simulink model "ADMIRE"  (R2021b)
settings: Solver=ode4  StartTime=0.0  StopTime=100  FixedStep=1e-2  RelTol=1e-3
undefined symbols (not defined in the file or in its folder): admireDB, Earth, WGS84
libraries: simulink_extras x112, simulink x27, aerolibutil x4, dspsigops x4, aerolibfltsims x3, sharedtransform x2, aerolibtransform2 x2, aerolibatmos2 x1, matrix_library x1, sharedutil x1, aerolibanimutils x1, vrlib x1
(part 9 of 15)

== system ADMIRE/Aircraft/Aerodynamics/CentripetalForceCoefficient/MachRegion1/Ccbde/Ccbde_ ==
  angleOfSideslip_deg : Inport
  dEI : Inport  Port=2
  angleOfAttack_deg : Inport  Port=3
  eieff : Inport  Port=4
  dEY : Inport  Port=5
  eoeff : Inport  Port=6
  Abs : Abs
  CCDEB_ALFA_DE_BETA : Lookup_n-D  NumberOfTableDimensions=3  BreakpointsForDimension1=admireDB.aerodata_asym_ext.CCDEB.breakpoints.ALFA  BreakpointsForDimension2=admireDB.aerodata_asym_ext.CCDEB.breakpoints.DE  BreakpointsForDimension3=admireDB.aerodata_asym_ext.CCDEB.breakpoints.BETA  Table=admireDB.aerodata_asym_ext.CCDEB.newTable  ExtrapMethod=Clip  InternalRulePriority=Speed  RndMeth=Simplest  InputSameDT=on
      settings: InputPortMap=u0,u1,u2
  CCDEB_ALFA_DE_BETA1 : Lookup_n-D  NumberOfTableDimensions=3  BreakpointsForDimension1=admireDB.aerodata_asym_ext.CCDEB.breakpoints.ALFA  BreakpointsForDimension2=admireDB.aerodata_asym_ext.CCDEB.breakpoints.DE  BreakpointsForDimension3=admireDB.aerodata_asym_ext.CCDEB.breakpoints.BETA  Table=admireDB.aerodata_asym_ext.CCDEB.newTable  ExtrapMethod=Clip  InternalRulePriority=Speed  RndMeth=Simplest  InputSameDT=on
      settings: InputPortMap=u0,u1,u2
  Product : Product  Inputs=**
  Product1 : Product  Inputs=**
  Product2 : Product  Inputs=**
  Sign : Signum
  Sum : Sum  Inputs=|++
  Ccbde : Outport
  wires:
  Abs/1 -> CCDEB_ALFA_DE_BETA1/3, CCDEB_ALFA_DE_BETA/3
  angleOfSideslip_deg/1 -> Sign/1, Abs/1
  Product2/1 -> Ccbde/1
  Sign/1 -> Product2/1
  Sum/1 -> Product2/2
  Product1/1 -> Sum/2
  Product/1 -> Sum/1
  CCDEB_ALFA_DE_BETA1/1 -> Product1/1
  eoeff/1 -> Product1/2
  dEY/1 -> CCDEB_ALFA_DE_BETA1/2
  CCDEB_ALFA_DE_BETA/1 -> Product/1
  eieff/1 -> Product/2
  dEI/1 -> CCDEB_ALFA_DE_BETA/2
  angleOfAttack_deg/1 -> CCDEB_ALFA_DE_BETA1/1, CCDEB_ALFA_DE_BETA/1

== system ADMIRE/Aircraft/Aerodynamics/CentripetalForceCoefficient/MachRegion1/Ccbdle/Ccbdle_ ==
  dLE : Inport
  angleOfSideslip_deg : Inport  Port=2
  angleOfAttack_deg : Inport  Port=3
  Abs : Abs
  CCDLEB_ALFA_BETA_DLE : Lookup_n-D  NumberOfTableDimensions=3  BreakpointsForDimension1=admireDB.aerodata_asym_ext.CCDLEB.breakpoints.ALFA  BreakpointsForDimension2=admireDB.aerodata_asym_ext.CCDLEB.breakpoints.BETA  BreakpointsForDimension3=admireDB.aerodata_asym_ext.CCDLEB.breakpoints.DLE  Table=admireDB.aerodata_asym_ext.CCDLEB.newTable  ExtrapMethod=Clip  InternalRulePriority=Speed  RndMeth=Simplest  InputSameDT=on
      settings: InputPortMap=u0,u1,u2
  Product : Product  Inputs=**
  Sign : Signum
  Ccbdle : Outport
  wires:
  Product/1 -> Ccbdle/1
  Sign/1 -> Product/2
  CCDLEB_ALFA_BETA_DLE/1 -> Product/1
  Abs/1 -> CCDLEB_ALFA_BETA_DLE/2
  angleOfAttack_deg/1 -> CCDLEB_ALFA_BETA_DLE/1
  angleOfSideslip_deg/1 -> Sign/1, Abs/1
  dLE/1 -> CCDLEB_ALFA_BETA_DLE/3

== system ADMIRE/Aircraft/Aerodynamics/CentripetalForceCoefficient/MachRegion1/Ccbdn/Ccbdn_ ==
  angleOfSideslip_deg : Inport
  dN : Inport  Port=2
  angleOfAttack_deg : Inport  Port=3
  Abs : Abs
  CCDNB_ALFA_DN_BETA : Lookup_n-D  NumberOfTableDimensions=3  BreakpointsForDimension1=admireDB.aerodata_asym_ext.CCDNB.breakpoints.ALFA  BreakpointsForDimension2=admireDB.aerodata_asym_ext.CCDNB.breakpoints.DN  BreakpointsForDimension3=admireDB.aerodata_asym_ext.CCDNB.breakpoints.BETA  Table=admireDB.aerodata_asym_ext.CCDNB.newTable  ExtrapMethod=Clip  InternalRulePriority=Speed  RndMeth=Simplest  InputSameDT=on
      settings: InputPortMap=u0,u1,u2
  Product : Product  Inputs=**
  Sign : Signum
  Ccbdn : Outport
  wires:
  Abs/1 -> CCDNB_ALFA_DN_BETA/3
  angleOfAttack_deg/1 -> CCDNB_ALFA_DN_BETA/1
  Product/1 -> Ccbdn/1
  Sign/1 -> Product/2
  CCDNB_ALFA_DN_BETA/1 -> Product/1
  dN/1 -> CCDNB_ALFA_DN_BETA/2
  angleOfSideslip_deg/1 -> Abs/1, Sign/1

== system ADMIRE/Aircraft/Aerodynamics/CentripetalForceCoefficient/MachRegion1/Ccbeta/Ccbeta_ ==
  angleOfSideslip_deg : Inport
  angleOfAttack_deg : Inport  Port=2
  qacorr : Inport  Port=3
  mach_nd : Inport  Port=4
  Abs : Abs
  CCBAL_BETA_ALFA : Lookup_n-D  BreakpointsForDimension1=admireDB.aerodata_asym_ext.CCBAL.breakpoints.ALFA  BreakpointsForDimension2=admireDB.aerodata_asym_ext.CCBAL.breakpoints.BETA  BreakpointsForDimension3=[5, 7]  Table=admireDB.aerodata_asym_ext.CCBAL.newTable  ExtrapMethod=Clip  InternalRulePriority=Speed  RndMeth=Simplest  InputSameDT=on
      settings: InputPortMap=u0,u1
  CCEB_QA_M : Lookup_n-D  BreakpointsForDimension1=admireDB.aerodata_asym_ext.CCEB.breakpoints.M  BreakpointsForDimension2=admireDB.aerodata_asym_ext.CCEB.breakpoints.QA  BreakpointsForDimension3=[5, 7]  Table=admireDB.aerodata_asym_ext.CCEB.newTable  ExtrapMethod=Clip  InternalRulePriority=Speed  RndMeth=Simplest  InputSameDT=on
      settings: InputPortMap=u0,u1
  Product : Product  Inputs=***
  Sign : Signum
  Ccbeta : Outport
  wires:
  Product/1 -> Ccbeta/1
  Sign/1 -> Product/1
  CCBAL_BETA_ALFA/1 -> Product/2
  CCEB_QA_M/1 -> Product/3
  Abs/1 -> CCBAL_BETA_ALFA/2
  angleOfSideslip_deg/1 -> Abs/1, Sign/1
  angleOfAttack_deg/1 -> CCBAL_BETA_ALFA/1
  qacorr/1 -> CCEB_QA_M/2
  mach_nd/1 -> CCEB_QA_M/1

== system ADMIRE/Aircraft/Aerodynamics/CentripetalForceCoefficient/MachRegion1/Ccbetad/Ccbetad_ ==
  angleOfAttack_deg : Inport
  betad : Inport  Port=2
  CCBDL_ALFA : Lookup_n-D  NumberOfTableDimensions=1  BreakpointsForDimension1=admireDB.aerodata_asym_ext.CCBDL.breakpoints.ALFA  BreakpointsForDimension3=[5, 7]  Table=admireDB.aerodata_asym_ext.CCBDL.newTable  ExtrapMethod=Clip  InternalRulePriority=Speed  RndMeth=Simplest  InputSameDT=on
  Product : Product
  Ccbetad : Outport
  wires:
  Product/1 -> Ccbetad/1
  betad/1 -> Product/2
  CCBDL_ALFA/1 -> Product/1
  angleOfAttack_deg/1 -> CCBDL_ALFA/1

== system ADMIRE/Aircraft/Aerodynamics/CentripetalForceCoefficient/MachRegion1/Ccblg/Ccblg_ ==
  dLG : Inport
  angleOfAttack_deg : Inport  Port=2
  angleOfSideslip_deg : Inport  Port=3
  CCBLST_NG_DOOR_ALFA : Lookup_n-D  BreakpointsForDimension1=admireDB.aerodata_asym_ext.CCBLST.breakpoints.ALFA  BreakpointsForDimension2=admireDB.aerodata_asym_ext.CCBLST.breakpoints.NG_DOOR  BreakpointsForDimension3=[5, 7]  Table=admireDB.aerodata_asym_ext.CCBLST.newTable  ExtrapMethod=Clip  InternalRulePriority=Speed  RndMeth=Simplest  InputSameDT=on
      settings: InputPortMap=u0,u1
  Degrees to Radians : simulink_extras/Transformations/Degrees to Radians
  Product : Product  Inputs=***
  Ccblg : Outport
  wires:
  Product/1 -> Ccblg/1
  Degrees to Radians/1 -> Product/2
  angleOfSideslip_deg/1 -> Degrees to Radians/1
  CCBLST_NG_DOOR_ALFA/1 -> Product/1
  dLG/1 -> Product/3, CCBLST_NG_DOOR_ALFA/2
  angleOfAttack_deg/1 -> CCBLST_NG_DOOR_ALFA/1

== system ADMIRE/Aircraft/Aerodynamics/CentripetalForceCoefficient/MachRegion1/Ccdai/Ccdai_ ==
  dAI : Inport
  angleOfAttack_deg : Inport  Port=2
  dEI : Inport  Port=3
  eieff : Inport  Port=4
  qacorr : Inport  Port=5
  mach_nd : Inport  Port=6
  Abs : Abs
  CCDAAL_DA_ALFA : Lookup_n-D  BreakpointsForDimension1=admireDB.aerodata_asym_ext.CCDAAL.breakpoints.ALFA  BreakpointsForDimension2=admireDB.aerodata_asym_ext.CCDAAL.breakpoints.DA  BreakpointsForDimension3=[5, 7]  Table=admireDB.aerodata_asym_ext.CCDAAL.newTable  ExtrapMethod=Clip  InternalRulePriority=Speed  RndMeth=Simplest  InputSameDT=on
      settings: InputPortMap=u0,u1
  CCDAL_DE_ALFA : Lookup_n-D  BreakpointsForDimension1=admireDB.aerodata_asym_ext.CCDAL.breakpoints.ALFA  BreakpointsForDimension2=admireDB.aerodata_asym_ext.CCDAL.breakpoints.DE  BreakpointsForDimension3=[5, 7]  Table=admireDB.aerodata_asym_ext.CCDAL.newTable  ExtrapMethod=Clip  InternalRulePriority=Speed  RndMeth=Simplest  InputSameDT=on
      settings: InputPortMap=u0,u1
  CCDAL_DE_ALFA_1 : Lookup_n-D  BreakpointsForDimension1=admireDB.aerodata_asym_ext.CCDAL.breakpoints.ALFA  BreakpointsForDimension2=admireDB.aerodata_asym_ext.CCDAL.breakpoints.DE  BreakpointsForDimension3=[5, 7]  Table=admireDB.aerodata_asym_ext.CCDAL.newTable  ExtrapMethod=Clip  InternalRulePriority=Speed  RndMeth=Simplest  InputSameDT=on
      settings: InputPortMap=u0,u1
  CCEDAI_QA_M : Lookup_n-D  BreakpointsForDimension1=admireDB.aerodata_asym_ext.CCEDAI.breakpoints.M  BreakpointsForDimension2=admireDB.aerodata_asym_ext.CCEDAI.breakpoints.QA  BreakpointsForDimension3=[5, 7]  Table=admireDB.aerodata_asym_ext.CCEDAI.newTable  ExtrapMethod=Clip  InternalRulePriority=Speed  RndMeth=Simplest  InputSameDT=on
      settings: InputPortMap=u0,u1
  Degrees to Radians : simulink_extras/Transformations/Degrees to Radians
  Product : Product  Inputs=**
  Product1 : Product  Inputs=**
  Product2 : Product  Inputs=3
  Sign : Signum
  Sum : Sum  Inputs=|++
  Sum1 : Sum  Inputs=|+-
  dE_cnst : Constant  Value=0.0
  Ccdai : Outport
  wires:
  Sum1/1 -> Product1/2
  Product2/1 -> Ccdai/1
  CCEDAI_QA_M/1 -> Product2/3
  qacorr/1 -> CCEDAI_QA_M/2
  mach_nd/1 -> CCEDAI_QA_M/1
  Sum/1 -> Product2/1
  eieff/1 -> Product2/2
  Product1/1 -> Sum/2
  Degrees to Radians/1 -> Product1/1
  CCDAL_DE_ALFA_1/1 -> Sum1/2
  CCDAL_DE_ALFA/1 -> Sum1/1
  angleOfAttack_deg/1 -> CCDAL_DE_ALFA/1, CCDAL_DE_ALFA_1/1, CCDAAL_DA_ALFA/1
  dEI/1 -> CCDAL_DE_ALFA/2
  dE_cnst/1 -> CCDAL_DE_ALFA_1/2
  Product/1 -> Sum/1
  Abs/1 -> CCDAAL_DA_ALFA/2
  Sign/1 -> Product/1
  CCDAAL_DA_ALFA/1 -> Product/2
  dAI/1 -> Sign/1, Abs/1, Degrees to Radians/1

== system ADMIRE/Aircraft/Aerodynamics/CentripetalForceCoefficient/MachRegion1/Ccdaib/Ccdaib_ ==
  angleOfAttack_deg : Inport
  dAI : Inport  Port=2
  angleOfSideslip_deg : Inport  Port=3
  eieff : Inport  Port=4
  Abs : Abs
  Abs1 : Abs
  Abs2 : Abs
  CCDABAL_ALFA : Lookup_n-D  NumberOfTableDimensions=1  BreakpointsForDimension1=admireDB.aerodata_asym_ext.CCDABAL.breakpoints.ALFA  BreakpointsForDimension3=[5, 7]  Table=admireDB.aerodata_asym_ext.CCDABAL.newTable  ExtrapMethod=Clip  InternalRulePriority=Speed  RndMeth=Simplest  InputSameDT=on
  Constant : Constant  Value=30
  Constant1 : Constant  Value=20
  Product : Product  Inputs=**/*/*
  Ccdaib : Outport
  wires:
  Abs2/1 -> CCDABAL_ALFA/1
  Constant1/1 -> Product/5
  Abs1/1 -> Product/4
  angleOfSideslip_deg/1 -> Abs1/1
  Constant/1 -> Product/3
  Abs/1 -> Product/2
  CCDABAL_ALFA/1 -> Product/1
  Product/1 -> Ccdaib/1
  angleOfAttack_deg/1 -> Abs2/1
  dAI/1 -> Abs/1
  eieff/1 -> Product/6

== system ADMIRE/Aircraft/Aerodynamics/CentripetalForceCoefficient/MachRegion1/Ccday/Ccday_ ==
  dAY : Inport
  angleOfAttack_deg : Inport  Port=2
  dEY : Inport  Port=3
  eoeff : Inport  Port=4
  qacorr : Inport  Port=5
  mach_nd : Inport  Port=6
  Abs : Abs
  CCDAAL_DA_ALFA : Lookup_n-D  BreakpointsForDimension1=admireDB.aerodata_asym_ext.CCDAAL.breakpoints.ALFA  BreakpointsForDimension2=admireDB.aerodata_asym_ext.CCDAAL.breakpoints.DA  BreakpointsForDimension3=[5, 7]  Table=admireDB.aerodata_asym_ext.CCDAAL.newTable  ExtrapMethod=Clip  InternalRulePriority=Speed  RndMeth=Simplest  InputSameDT=on
      settings: InputPortMap=u0,u1
  CCDAL_DE_ALFA : Lookup_n-D  BreakpointsForDimension1=admireDB.aerodata_asym_ext.CCDAL.breakpoints.ALFA  BreakpointsForDimension2=admireDB.aerodata_asym_ext.CCDAL.breakpoints.DE  BreakpointsForDimension3=[5, 7]  Table=admireDB.aerodata_asym_ext.CCDAL.newTable  ExtrapMethod=Clip  InternalRulePriority=Speed  RndMeth=Simplest  InputSameDT=on
      settings: InputPortMap=u0,u1
  CCDAL_DE_ALFA_1 : Lookup_n-D  BreakpointsForDimension1=admireDB.aerodata_asym_ext.CCDAL.breakpoints.ALFA  BreakpointsForDimension2=admireDB.aerodata_asym_ext.CCDAL.breakpoints.DE  BreakpointsForDimension3=[5, 7]  Table=admireDB.aerodata_asym_ext.CCDAL.newTable  ExtrapMethod=Clip  InternalRulePriority=Speed  RndMeth=Simplest  InputSameDT=on
      settings: InputPortMap=u0,u1
  CCEDAY_QA_M : Lookup_n-D  BreakpointsForDimension1=admireDB.aerodata_asym_ext.CCEDAY.breakpoints.M  BreakpointsForDimension2=admireDB.aerodata_asym_ext.CCEDAY.breakpoints.QA  BreakpointsForDimension3=[5, 7]  Table=admireDB.aerodata_asym_ext.CCEDAY.newTable  ExtrapMethod=Clip  InternalRulePriority=Speed  RndMeth=Simplest  InputSameDT=on
      settings: InputPortMap=u0,u1
  Degrees to Radians : simulink_extras/Transformations/Degrees to Radians
  Product : Product  Inputs=**
  Product1 : Product  Inputs=**
  Product2 : Product
  Product3 : Product
  Sign : Signum
  Sum : Sum  Inputs=|++
  Sum1 : Sum  Inputs=|++
  Sum2 : Sum  Inputs=|+-
  dE_cnst : Constant  Value=0.0
  Ccday : Outport
  wires:
  Sum2/1 -> Product1/2
  CCDAL_DE_ALFA_1/1 -> Sum2/2
  CCDAL_DE_ALFA/1 -> Sum2/1
  CCEDAY_QA_M/1 -> Product3/2
  Product2/1 -> Sum1/1
  Sum1/1 -> Ccday/1
  dAY/1 -> Abs/1, Degrees to Radians/1, Sign/1
  CCDAAL_DA_ALFA/1 -> Product/2
  Sign/1 -> Product/1
  Abs/1 -> CCDAAL_DA_ALFA/2
  Product/1 -> Sum/1
  dE_cnst/1 -> CCDAL_DE_ALFA_1/2
  dEY/1 -> CCDAL_DE_ALFA/2
  angleOfAttack_deg/1 -> CCDAL_DE_ALFA/1, CCDAL_DE_ALFA_1/1, CCDAAL_DA_ALFA/1
  Degrees to Radians/1 -> Product1/1, Product3/1
  Product1/1 -> Sum/2
  eoeff/1 -> Product2/2
  Sum/1 -> Product2/1
  mach_nd/1 -> CCEDAY_QA_M/1
  qacorr/1 -> CCEDAY_QA_M/2
  Product3/1 -> Sum1/2

== system ADMIRE/Aircraft/Aerodynamics/CentripetalForceCoefficient/MachRegion1/Ccdayb/Ccdayb_ ==
  angleOfAttack_deg : Inport
  dAY : Inport  Port=2
  angleOfSideslip_deg : Inport  Port=3
  eoeff : Inport  Port=4
  Abs : Abs
  Abs1 : Abs
  Abs2 : Abs
  CCDABAL_ALFA : Lookup_n-D  NumberOfTableDimensions=1  BreakpointsForDimension1=admireDB.aerodata_asym_ext.CCDABAL.breakpoints.ALFA  BreakpointsForDimension3=[5, 7]  Table=admireDB.aerodata_asym_ext.CCDABAL.newTable  ExtrapMethod=Clip  InternalRulePriority=Speed  RndMeth=Simplest  InputSameDT=on
  Constant : Constant  Value=30
  Constant1 : Constant  Value=20
  Product : Product  Inputs=**/*/*
  Ccdayb : Outport
  wires:
  eoeff/1 -> Product/6
  dAY/1 -> Abs/1
  angleOfAttack_deg/1 -> Abs2/1
  Product/1 -> Ccdayb/1
  CCDABAL_ALFA/1 -> Product/1
  Abs/1 -> Product/2
  Constant/1 -> Product/3
  angleOfSideslip_deg/1 -> Abs1/1
  Abs1/1 -> Product/4
  Constant1/1 -> Product/5
  Abs2/1 -> CCDABAL_ALFA/1

== system ADMIRE/Aircraft/Aerodynamics/CentripetalForceCoefficient/MachRegion1/Ccdna/Ccdna_ ==
  dNE : Inport
  angleOfAttack_deg : Inport  Port=2
  dNA : Inport  Port=3
  CCDNAAL_DNE_ALFA : Lookup_n-D  BreakpointsForDimension1=admireDB.aerodata_asym_ext.CCDNAAL.breakpoints.ALFA  BreakpointsForDimension2=admireDB.aerodata_asym_ext.CCDNAAL.breakpoints.DNE  BreakpointsForDimension3=[5, 7]  Table=admireDB.aerodata_asym_ext.CCDNAAL.newTable  ExtrapMethod=Clip  InternalRulePriority=Speed  RndMeth=Simplest  InputSameDT=on
      settings: InputPortMap=u0,u1
  Degrees to Radians : simulink_extras/Transformations/Degrees to Radians
  Product : Product
  Ccdna : Outport
  wires:
  Product/1 -> Ccdna/1
  Degrees to Radians/1 -> Product/2
  CCDNAAL_DNE_ALFA/1 -> Product/1
  dNA/1 -> Degrees to Radians/1
  dNE/1 -> CCDNAAL_DNE_ALFA/2
  angleOfAttack_deg/1 -> CCDNAAL_DNE_ALFA/1

== system ADMIRE/Aircraft/Aerodynamics/CentripetalForceCoefficient/MachRegion1/Ccdr/Ccdr_ ==
  angleOfAttack_deg : Inport
  dR : Inport  Port=2
  angleOfSideslip_deg : Inport  Port=3
  qacorr : Inport  Port=4
  mach_nd : Inport  Port=5
  Abs : Abs
  CCBDRAL_ALFA_DR_BETA : Lookup_n-D  NumberOfTableDimensions=3  BreakpointsForDimension1=admireDB.aerodata_asym_ext.CCBDRAL.breakpoints.ALFA  BreakpointsForDimension2=admireDB.aerodata_asym_ext.CCBDRAL.breakpoints.DR  BreakpointsForDimension3=admireDB.aerodata_asym_ext.CCBDRAL.breakpoints.BETA  Table=admireDB.aerodata_asym_ext.CCBDRAL.newTable  ExtrapMethod=Clip  InternalRulePriority=Speed  RndMeth=Simplest  InputSameDT=on
      settings: InputPortMap=u0,u1,u2
  CCEDR_QA_M : Lookup_n-D  BreakpointsForDimension1=admireDB.aerodata_asym_ext.CCEDR.breakpoints.M  BreakpointsForDimension2=admireDB.aerodata_asym_ext.CCEDR.breakpoints.QA  BreakpointsForDimension3=[5, 7]  Table=admireDB.aerodata_asym_ext.CCEDR.newTable  ExtrapMethod=Clip  InternalRulePriority=Speed  RndMeth=Simplest  InputSameDT=on
      settings: InputPortMap=u0,u1
  Product : Product  Inputs=**
  Ccdr : Outport
  wires:
  Abs/1 -> CCBDRAL_ALFA_DR_BETA/3
  angleOfAttack_deg/1 -> CCBDRAL_ALFA_DR_BETA/1
  Product/1 -> Ccdr/1
  CCEDR_QA_M/1 -> Product/2
  CCBDRAL_ALFA_DR_BETA/1 -> Product/1
  angleOfSideslip_deg/1 -> Abs/1
  dR/1 -> CCBDRAL_ALFA_DR_BETA/2
  qacorr/1 -> CCEDR_QA_M/2
  mach_nd/1 -> CCEDR_QA_M/1

== system ADMIRE/Aircraft/Aerodynamics/CentripetalForceCoefficient/MachRegion1/Ccp/Ccp_ ==
  angleOfAttack_deg : Inport
  pc : Inport  Port=2
  CCPAL_ALFA : Lookup_n-D  NumberOfTableDimensions=1  BreakpointsForDimension1=admireDB.aerodata_asym_ext.CCPAL.breakpoints.ALFA  BreakpointsForDimension3=[5, 7]  Table=admireDB.aerodata_asym_ext.CCPAL.newTable  ExtrapMethod=Clip  InternalRulePriority=Speed  RndMeth=Simplest  InputSameDT=on
  Product : Product
  Ccp : Outport
  wires:
  angleOfAttack_deg/1 -> CCPAL_ALFA/1
  CCPAL_ALFA/1 -> Product/1
  pc/1 -> Product/2
  Product/1 -> Ccp/1

== system ADMIRE/Aircraft/Aerodynamics/CentripetalForceCoefficient/MachRegion1/Ccpbeta/Ccpbeta_ ==
  angleOfSideslip_deg : Inport
  pc : Inport  Port=2
  angleOfAttack_deg : Inport  Port=3
  Abs : Abs
  CCPBA_BETA_ALFA : Lookup_n-D  BreakpointsForDimension1=admireDB.aerodata_asym_ext.CCPBA.breakpoints.ALFA  BreakpointsForDimension2=admireDB.aerodata_asym_ext.CCPBA.breakpoints.BETA  BreakpointsForDimension3=[5, 7]  Table=admireDB.aerodata_asym_ext.CCPBA.newTable  ExtrapMethod=Clip  InternalRulePriority=Speed  RndMeth=Simplest  InputSameDT=on
      settings: InputPortMap=u0,u1
  Product : Product
  Ccpbeta : Outport
  wires:
  Abs/1 -> CCPBA_BETA_ALFA/2
  angleOfSideslip_deg/1 -> Abs/1
  angleOfAttack_deg/1 -> CCPBA_BETA_ALFA/1
  Product/1 -> Ccpbeta/1
  pc/1 -> Product/2
  CCPBA_BETA_ALFA/1 -> Product/1

== system ADMIRE/Aircraft/Aerodynamics/CentripetalForceCoefficient/MachRegion1/Ccr/Ccr_ ==
  dN : Inport
  angleOfAttack_deg : Inport  Port=2
  rc : Inport  Port=3
  CCRAL_DNV_ALFA : Lookup_n-D  BreakpointsForDimension1=admireDB.aerodata_asym_ext.CCRAL.breakpoints.ALFA  BreakpointsForDimension2=admireDB.aerodata_asym_ext.CCRAL.breakpoints.DNV  BreakpointsForDimension3=[5, 7]  Table=admireDB.aerodata_asym_ext.CCRAL.newTable  ExtrapMethod=Clip  InternalRulePriority=Speed  RndMeth=Simplest  InputSameDT=on
      settings: InputPortMap=u0,u1
  Product : Product
  Ccr : Outport
  wires:
  CCRAL_DNV_ALFA/1 -> Product/1
  dN/1 -> CCRAL_DNV_ALFA/2
  angleOfAttack_deg/1 -> CCRAL_DNV_ALFA/1
  rc/1 -> Product/2
  Product/1 -> Ccr/1

== system ADMIRE/Aircraft/Aerodynamics/CentripetalForceCoefficient/MachRegion1/Ccrbeta/Ccrbeta_ ==
  angleOfSideslip_deg : Inport
  angleOfAttack_deg : Inport  Port=2
  rc : Inport  Port=3
  Abs : Abs
  Abs1 : Abs
  CCRBA_BETA_ALFA : Lookup_n-D  BreakpointsForDimension1=admireDB.aerodata_asym_ext.CCRBA.breakpoints.ALFA  BreakpointsForDimension2=admireDB.aerodata_asym_ext.CCRBA.breakpoints.BETA  BreakpointsForDimension3=[5, 7]  Table=admireDB.aerodata_asym_ext.CCRBA.newTable  ExtrapMethod=Clip  InternalRulePriority=Speed  RndMeth=Simplest  InputSameDT=on
      settings: InputPortMap=u0,u1
  Product : Product
  Ccrbeta : Outport
  wires:
  Abs1/1 -> CCRBA_BETA_ALFA/1
  Abs/1 -> CCRBA_BETA_ALFA/2
  angleOfSideslip_deg/1 -> Abs/1
  angleOfAttack_deg/1 -> Abs1/1
  Product/1 -> Ccrbeta/1
  rc/1 -> Product/2
  CCRBA_BETA_ALFA/1 -> Product/1

== system ADMIRE/Aircraft/Aerodynamics/CentripetalForceCoefficient/MachRegion2/Ccbcai/Ccbcai_ ==
  cai : Inport
  angleOfAttack_deg : Inport  Port=2
  angleOfSideslip_deg : Inport  Port=3
  CCBCAI_CAI_ALFA : Lookup_n-D  BreakpointsForDimension1=admireDB.aerodata_asym_ext.CCBCAI.breakpoints.ALFA  BreakpointsForDimension2=admireDB.aerodata_asym_ext.CCBCAI.breakpoints.CAI  BreakpointsForDimension3=[5, 7]  Table=admireDB.aerodata_asym_ext.CCBCAI.newTable  ExtrapMethod=Clip  InternalRulePriority=Speed  RndMeth=Simplest  InputSameDT=on
      settings: InputPortMap=u0,u1
  Degrees to Radians : simulink_extras/Transformations/Degrees to Radians
  Product : Product
  Ccbcai : Outport
  wires:
  Product/1 -> Ccbcai/1
  cai/1 -> CCBCAI_CAI_ALFA/2
  angleOfAttack_deg/1 -> CCBCAI_CAI_ALFA/1
  angleOfSideslip_deg/1 -> Degrees to Radians/1
  Degrees to Radians/1 -> Product/2
  CCBCAI_CAI_ALFA/1 -> Product/1

== system ADMIRE/Aircraft/Aerodynamics/CentripetalForceCoefficient/MachRegion2/Ccbde/Ccbde_ ==
  angleOfAttack_deg : Inport
  dEI : Inport  Port=2
  angleOfSideslip_deg : Inport  Port=3
  eieff : Inport  Port=4
  dEY : Inport  Port=5
  eoeff : Inport  Port=6
  Abs : Abs
  CCDEB_ALFA_DE_BETA : Lookup_n-D  NumberOfTableDimensions=3  BreakpointsForDimension1=admireDB.aerodata_asym_ext.CCDEB.breakpoints.ALFA  BreakpointsForDimension2=admireDB.aerodata_asym_ext.CCDEB.breakpoints.DE  BreakpointsForDimension3=admireDB.aerodata_asym_ext.CCDEB.breakpoints.BETA  Table=admireDB.aerodata_asym_ext.CCDEB.newTable  ExtrapMethod=Clip  InternalRulePriority=Speed  RndMeth=Simplest  InputSameDT=on
      settings: InputPortMap=u0,u1,u2
  CCDEB_ALFA_DE_BETA1 : Lookup_n-D  NumberOfTableDimensions=3  BreakpointsForDimension1=admireDB.aerodata_asym_ext.CCDEB.breakpoints.ALFA  BreakpointsForDimension2=admireDB.aerodata_asym_ext.CCDEB.breakpoints.DE  BreakpointsForDimension3=admireDB.aerodata_asym_ext.CCDEB.breakpoints.BETA  Table=admireDB.aerodata_asym_ext.CCDEB.newTable  ExtrapMethod=Clip  InternalRulePriority=Speed  RndMeth=Simplest  InputSameDT=on
      settings: InputPortMap=u0,u1,u2
  Product : Product
  Product1 : Product
  Product2 : Product
  Sign : Signum
  Sum : Sum  Inputs=|++
  Ccbde : Outport
  wires:
  Product2/1 -> Ccbde/1
  angleOfAttack_deg/1 -> CCDEB_ALFA_DE_BETA/1, CCDEB_ALFA_DE_BETA1/1
  dEI/1 -> CCDEB_ALFA_DE_BETA/2
  eieff/1 -> Product/2
  CCDEB_ALFA_DE_BETA/1 -> Product/1
  dEY/1 -> CCDEB_ALFA_DE_BETA1/2
  eoeff/1 -> Product1/2
  CCDEB_ALFA_DE_BETA1/1 -> Product1/1
  Product/1 -> Sum/1
  Product1/1 -> Sum/2
  Sum/1 -> Product2/1
  Sign/1 -> Product2/2
  angleOfSideslip_deg/1 -> Sign/1, Abs/1
  Abs/1 -> CCDEB_ALFA_DE_BETA/3, CCDEB_ALFA_DE_BETA1/3

== system ADMIRE/Aircraft/Aerodynamics/CentripetalForceCoefficient/MachRegion2/Ccbdle/Ccbdle_ ==
  angleOfAttack_deg : Inport
  angleOfSideslip_deg : Inport  Port=2
  dLE : Inport  Port=3
  tflow : Inport  Port=4
  tfhigh : Inport  Port=5
  Abs : Abs
  CCBDLE_M_ALFA : Lookup_n-D  BreakpointsForDimension1=admireDB.aerodata_asym_ext.CCBDLE.breakpoints.ALFA  BreakpointsForDimension2=admireDB.aerodata_asym_ext.CCBDLE.breakpoints.M  BreakpointsForDimension3=[5, 7]  Table=admireDB.aerodata_asym_ext.CCBDLE.newTable  ExtrapMethod=Clip  InternalRulePriority=Speed  RndMeth=Simplest  InputSameDT=on
      settings: InputPortMap=u0,u1
  CCDLEB_ALFA_BETA_DLE : Lookup_n-D  NumberOfTableDimensions=3  BreakpointsForDimension1=admireDB.aerodata_asym_ext.CCDLEB.breakpoints.ALFA  BreakpointsForDimension2=admireDB.aerodata_asym_ext.CCDLEB.breakpoints.BETA  BreakpointsForDimension3=admireDB.aerodata_asym_ext.CCDLEB.breakpoints.DLE  Table=admireDB.aerodata_asym_ext.CCDLEB.newTable  ExtrapMethod=Clip  InternalRulePriority=Speed  RndMeth=Simplest  InputSameDT=on
      settings: InputPortMap=u0,u1,u2
  Constant : Constant  Value=0.5
  Constant1 : Constant  Value=1/27
  Degrees to Radians : simulink_extras/Transformations/Degrees to Radians
  Product : Product  Inputs=3
  Product1 : Product  Inputs=5
  Sign : Signum
  Sum : Sum  Inputs=|++
  Ccbdle : Outport
  wires:
  Constant/1 -> CCBDLE_M_ALFA/2
  angleOfSideslip_deg/1 -> Degrees to Radians/1, Sign/1, Abs/1
  Abs/1 -> CCDLEB_ALFA_BETA_DLE/2
  tflow/1 -> Product/2
  CCDLEB_ALFA_BETA_DLE/1 -> Product/1
  Sign/1 -> Product/3
  Product/1 -> Sum/1
  angleOfAttack_deg/1 -> CCDLEB_ALFA_BETA_DLE/1, CCBDLE_M_ALFA/1
  Degrees to Radians/1 -> Product1/1
  CCBDLE_M_ALFA/1 -> Product1/4
  tfhigh/1 -> Product1/5
  Constant1/1 -> Product1/3
  dLE/1 -> CCDLEB_ALFA_BETA_DLE/3, Product1/2
  Product1/1 -> Sum/2
  Sum/1 -> Ccbdle/1

== system ADMIRE/Aircraft/Aerodynamics/CentripetalForceCoefficient/MachRegion2/Ccbdn/Ccbdn_ ==
  angleOfAttack_deg : Inport
  dN : Inport  Port=2
  angleOfSideslip_deg : Inport  Port=3
  Abs : Abs
  CCDNB_ALFA_DN_BETA : Lookup_n-D  NumberOfTableDimensions=3  BreakpointsForDimension1=admireDB.aerodata_asym_ext.CCDNB.breakpoints.ALFA  BreakpointsForDimension2=admireDB.aerodata_asym_ext.CCDNB.breakpoints.DN  BreakpointsForDimension3=admireDB.aerodata_asym_ext.CCDNB.breakpoints.BETA  Table=admireDB.aerodata_asym_ext.CCDNB.newTable  ExtrapMethod=Clip  InternalRulePriority=Speed  RndMeth=Simplest  InputSameDT=on
      settings: InputPortMap=u0,u1,u2
  Product : Product
  Sign : Signum
  Ccbdn : Outport
  wires:
  angleOfAttack_deg/1 -> CCDNB_ALFA_DN_BETA/1
  dN/1 -> CCDNB_ALFA_DN_BETA/2
  angleOfSideslip_deg/1 -> Sign/1, Abs/1
  Abs/1 -> CCDNB_ALFA_DN_BETA/3
  CCDNB_ALFA_DN_BETA/1 -> Product/1
  Sign/1 -> Product/2
  Product/1 -> Ccbdn/1

== system ADMIRE/Aircraft/Aerodynamics/CentripetalForceCoefficient/MachRegion2/Ccbeta/Ccbeta_ ==
  angleOfSideslip_deg : Inport
  angleOfAttack_deg : Inport  Port=2
  tflow : Inport  Port=3
  tfhigh : Inport  Port=4
  qacorr : Inport  Port=5
  mach_nd : Inport  Port=6
  Abs : Abs
  CCBAL_BETA_ALFA : Lookup_n-D  BreakpointsForDimension1=admireDB.aerodata_asym_ext.CCBAL.breakpoints.ALFA  BreakpointsForDimension2=admireDB.aerodata_asym_ext.CCBAL.breakpoints.BETA  BreakpointsForDimension3=[5, 7]  Table=admireDB.aerodata_asym_ext.CCBAL.newTable  ExtrapMethod=Clip  InternalRulePriority=Speed  RndMeth=Simplest  InputSameDT=on
      settings: InputPortMap=u0,u1
  CCBMA_M_ALFA : Lookup_n-D  BreakpointsForDimension1=admireDB.aerodata_asym_ext.CCBMA.breakpoints.ALFA  BreakpointsForDimension2=admireDB.aerodata_asym_ext.CCBMA.breakpoints.M  BreakpointsForDimension3=[5, 7]  Table=admireDB.aerodata_asym_ext.CCBMA.newTable  ExtrapMethod=Clip  InternalRulePriority=Speed  RndMeth=Simplest  InputSameDT=on
      settings: InputPortMap=u0,u1
  CCEB_QA_M : Lookup_n-D  BreakpointsForDimension1=admireDB.aerodata_asym_ext.CCEB.breakpoints.M  BreakpointsForDimension2=admireDB.aerodata_asym_ext.CCEB.breakpoints.QA  BreakpointsForDimension3=[5, 7]  Table=admireDB.aerodata_asym_ext.CCEB.newTable  ExtrapMethod=Clip  InternalRulePriority=Speed  RndMeth=Simplest  InputSameDT=on
      settings: InputPortMap=u0,u1
  Degrees to Radians : simulink_extras/Transformations/Degrees to Radians
  Product : Product  Inputs=3
  Product1 : Product  Inputs=3
  Product2 : Product
  Sign : Signum
  Sum : Sum  Inputs=|++
  mach_cnst : Constant  Value=0.5
  CCbeta : Outport
  wires:
  mach_cnst/1 -> CCBMA_M_ALFA/2
  angleOfSideslip_deg/1 -> Abs/1, Degrees to Radians/1, Sign/1
  angleOfAttack_deg/1 -> CCBAL_BETA_ALFA/1, CCBMA_M_ALFA/1
  CCBAL_BETA_ALFA/1 -> Product/1  "CCBAL"
  Sign/1 -> Product/3
  tflow/1 -> Product/2
  Abs/1 -> CCBAL_BETA_ALFA/2
  mach_nd/1 -> CCEB_QA_M/1
  CCBMA_M_ALFA/1 -> Product1/3
  tfhigh/1 -> Product1/2
  Degrees to Radians/1 -> Product1/1
  Product/1 -> Sum/1
  Product1/1 -> Sum/2
  qacorr/1 -> CCEB_QA_M/2
  CCEB_QA_M/1 -> Product2/2
  Product2/1 -> CCbeta/1
  Sum/1 -> Product2/1

== system ADMIRE/Aircraft/Aerodynamics/CentripetalForceCoefficient/MachRegion2/Ccbetad/CCbetad_ ==
  angleOfAttack_deg : Inport
  tflow : Inport  Port=2
  betad : Inport  Port=3
  tfhigh : Inport  Port=4
  CCBDH_ALFA_M : Lookup_n-D  BreakpointsForDimension1=admireDB.aerodata_asym_ext.CCBDH.breakpoints.M  BreakpointsForDimension2=admireDB.aerodata_asym_ext.CCBDH.breakpoints.ALFA  BreakpointsForDimension3=[5, 7]  Table=admireDB.aerodata_asym_ext.CCBDH.newTable  ExtrapMethod=Clip  InternalRulePriority=Speed  RndMeth=Simplest  InputSameDT=on
      settings: InputPortMap=u0,u1
  CCBDL_ALFA : Lookup_n-D  NumberOfTableDimensions=1  BreakpointsForDimension1=admireDB.aerodata_asym_ext.CCBDL.breakpoints.ALFA  BreakpointsForDimension3=[5, 7]  Table=admireDB.aerodata_asym_ext.CCBDL.newTable  ExtrapMethod=Clip  InternalRulePriority=Speed  RndMeth=Simplest  InputSameDT=on
  Constant : Constant  Value=0.5
  Product : Product
  Product1 : Product
  Product2 : Product
  Sum : Sum  Inputs=|++
  CCbetad : Outport
  wires:
  Product2/1 -> CCbetad/1
  angleOfAttack_deg/1 -> CCBDL_ALFA/1, CCBDH_ALFA_M/2
  tflow/1 -> Product/2
  CCBDL_ALFA/1 -> Product/1
  Product/1 -> Sum/1
  Constant/1 -> CCBDH_ALFA_M/1
  CCBDH_ALFA_M/1 -> Product1/2
  tfhigh/1 -> Product1/1
  Product1/1 -> Sum/2
  Sum/1 -> Product2/1
  betad/1 -> Product2/2

== system ADMIRE/Aircraft/Aerodynamics/CentripetalForceCoefficient/MachRegion2/Ccblg/Ccblg_ ==
  ldg : Inport
  angleOfAttack_deg : Inport  Port=2
  angleOfSideslip_deg : Inport  Port=3
  CCBLST_NG_DOOR_ALFA : Lookup_n-D  BreakpointsForDimension1=admireDB.aerodata_asym_ext.CCBLST.breakpoints.ALFA  BreakpointsForDimension2=admireDB.aerodata_asym_ext.CCBLST.breakpoints.NG_DOOR  BreakpointsForDimension3=[5, 7]  Table=admireDB.aerodata_asym_ext.CCBLST.newTable  ExtrapMethod=Clip  InternalRulePriority=Speed  RndMeth=Simplest  InputSameDT=on
      settings: InputPortMap=u0,u1
  Degrees to Radians : simulink_extras/Transformations/Degrees to Radians
  Product : Product  Inputs=3
  Ccblg : Outport
  wires:
  Product/1 -> Ccblg/1
  angleOfAttack_deg/1 -> CCBLST_NG_DOOR_ALFA/1
  ldg/1 -> CCBLST_NG_DOOR_ALFA/2, Product/1
  angleOfSideslip_deg/1 -> Degrees to Radians/1
  CCBLST_NG_DOOR_ALFA/1 -> Product/2
  Degrees to Radians/1 -> Product/3

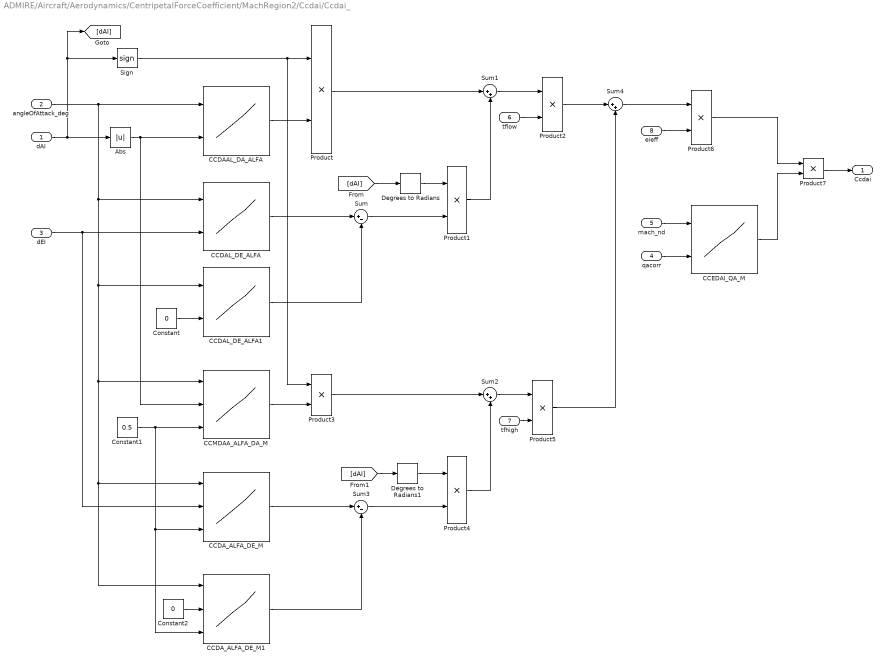
== system ADMIRE/Aircraft/Aerodynamics/CentripetalForceCoefficient/MachRegion2/Ccdai/Ccdai_ ==
  dAI : Inport
  angleOfAttack_deg : Inport  Port=2
  dEI : Inport  Port=3
  qacorr : Inport  Port=4
  mach_nd : Inport  Port=5
  tflow : Inport  Port=6
  tfhigh : Inport  Port=7
  eieff : Inport  Port=8
  Abs : Abs
  CCDAAL_DA_ALFA : Lookup_n-D  BreakpointsForDimension1=admireDB.aerodata_asym_ext.CCDAAL.breakpoints.ALFA  BreakpointsForDimension2=admireDB.aerodata_asym_ext.CCDAAL.breakpoints.DA  BreakpointsForDimension3=[5, 7]  Table=admireDB.aerodata_asym_ext.CCDAAL.newTable  ExtrapMethod=Clip  InternalRulePriority=Speed  RndMeth=Simplest  InputSameDT=on
      settings: InputPortMap=u0,u1
  CCDAL_DE_ALFA : Lookup_n-D  BreakpointsForDimension1=admireDB.aerodata_asym_ext.CCDAL.breakpoints.ALFA  BreakpointsForDimension2=admireDB.aerodata_asym_ext.CCDAL.breakpoints.DE  BreakpointsForDimension3=[5, 7]  Table=admireDB.aerodata_asym_ext.CCDAL.newTable  ExtrapMethod=Clip  InternalRulePriority=Speed  RndMeth=Simplest  InputSameDT=on
      settings: InputPortMap=u0,u1
  CCDAL_DE_ALFA1 : Lookup_n-D  BreakpointsForDimension1=admireDB.aerodata_asym_ext.CCDAL.breakpoints.ALFA  BreakpointsForDimension2=admireDB.aerodata_asym_ext.CCDAL.breakpoints.DE  BreakpointsForDimension3=[5, 7]  Table=admireDB.aerodata_asym_ext.CCDAL.newTable  ExtrapMethod=Clip  InternalRulePriority=Speed  RndMeth=Simplest  InputSameDT=on
      settings: InputPortMap=u0,u1
  CCDA_ALFA_DE_M : Lookup_n-D  NumberOfTableDimensions=3  BreakpointsForDimension1=admireDB.aerodata_asym_ext.CCDA.breakpoints.ALFA  BreakpointsForDimension2=admireDB.aerodata_asym_ext.CCDA.breakpoints.DE  BreakpointsForDimension3=admireDB.aerodata_asym_ext.CCDA.breakpoints.M  Table=admireDB.aerodata_asym_ext.CCDA.newTable  ExtrapMethod=Clip  InternalRulePriority=Speed  RndMeth=Simplest  InputSameDT=on
      settings: InputPortMap=u0,u1,u2
  CCDA_ALFA_DE_M1 : Lookup_n-D  NumberOfTableDimensions=3  BreakpointsForDimension1=admireDB.aerodata_asym_ext.CCDA.breakpoints.ALFA  BreakpointsForDimension2=admireDB.aerodata_asym_ext.CCDA.breakpoints.DE  BreakpointsForDimension3=admireDB.aerodata_asym_ext.CCDA.breakpoints.M  Table=admireDB.aerodata_asym_ext.CCDA.newTable  ExtrapMethod=Clip  InternalRulePriority=Speed  RndMeth=Simplest  InputSameDT=on
      settings: InputPortMap=u0,u1,u2
  CCEDAI_QA_M : Lookup_n-D  BreakpointsForDimension1=admireDB.aerodata_asym_ext.CCEDAI.breakpoints.M  BreakpointsForDimension2=admireDB.aerodata_asym_ext.CCEDAI.breakpoints.QA  BreakpointsForDimension3=[5, 7]  Table=admireDB.aerodata_asym_ext.CCEDAI.newTable  ExtrapMethod=Clip  InternalRulePriority=Speed  RndMeth=Simplest  InputSameDT=on
      settings: InputPortMap=u0,u1
  CCMDAA_ALFA_DA_M : Lookup_n-D  NumberOfTableDimensions=3  BreakpointsForDimension1=admireDB.aerodata_asym_ext.CCMDAA.breakpoints.ALFA  BreakpointsForDimension2=admireDB.aerodata_asym_ext.CCMDAA.breakpoints.DA  BreakpointsForDimension3=admireDB.aerodata_asym_ext.CCMDAA.breakpoints.M  Table=admireDB.aerodata_asym_ext.CCMDAA.newTable  ExtrapMethod=Clip  InternalRulePriority=Speed  RndMeth=Simplest  InputSameDT=on
      settings: InputPortMap=u0,u1,u2
  Constant : Constant  Value=0
  Constant1 : Constant  Value=0.5
  Constant2 : Constant  Value=0
  Degrees to Radians : simulink_extras/Transformations/Degrees to Radians
  Degrees to Radians1 : simulink_extras/Transformations/Degrees to Radians
  Product{,1..7} (8 alike) : Product
  Sign : Signum
  Sum : Sum  Inputs=|+-
  Sum1 : Sum  Inputs=|++
  Sum2 : Sum  Inputs=|++
  Sum3 : Sum  Inputs=|+-
  Sum4 : Sum  Inputs=|++
  Ccdai : Outport
  wires:
  CCDA_ALFA_DE_M1/1 -> Sum3/2
  Constant2/1 -> CCDA_ALFA_DE_M1/2
  CCDAL_DE_ALFA1/1 -> Sum/2
  Constant/1 -> CCDAL_DE_ALFA1/2
  dEI/1 -> CCDA_ALFA_DE_M/2, CCDAL_DE_ALFA/2
  angleOfAttack_deg/1 -> CCDAAL_DA_ALFA/1, CCDAL_DE_ALFA/1, CCDAL_DE_ALFA1/1, CCDA_ALFA_DE_M1/1, CCDA_ALFA_DE_M/1, CCMDAA_ALFA_DA_M/1
  dAI/1 -> Abs/1, [dAI], Sign/1
  CCDAAL_DA_ALFA/1 -> Product/2
  Sign/1 -> Product/1, Product3/1
  CCDAL_DE_ALFA/1 -> Sum/1
  [dAI] -> Degrees to Radians/1
  Degrees to Radians/1 -> Product1/1
  Sum/1 -> Product1/2
  Product/1 -> Sum1/1
  Product1/1 -> Sum1/2
  Sum1/1 -> Product2/1
  tflow/1 -> Product2/2
  Abs/1 -> CCMDAA_ALFA_DA_M/2, CCDAAL_DA_ALFA/2
  Constant1/1 -> CCDA_ALFA_DE_M1/3, CCDA_ALFA_DE_M/3, CCMDAA_ALFA_DA_M/3
  CCMDAA_ALFA_DA_M/1 -> Product3/2
  Product3/1 -> Sum2/1
  Sum3/1 -> Product4/2
  CCDA_ALFA_DE_M/1 -> Sum3/1
  [dAI] -> Degrees to Radians1/1
  Degrees to Radians1/1 -> Product4/1
  Product4/1 -> Sum2/2
  Sum2/1 -> Product5/1
  tfhigh/1 -> Product5/2
  Product2/1 -> Sum4/1
  Product5/1 -> Sum4/2
  eieff/1 -> Product6/2
  Sum4/1 -> Product6/1
  Product6/1 -> Product7/1
  mach_nd/1 -> CCEDAI_QA_M/1
  qacorr/1 -> CCEDAI_QA_M/2
  CCEDAI_QA_M/1 -> Product7/2
  Product7/1 -> Ccdai/1

== system ADMIRE/Aircraft/Aerodynamics/CentripetalForceCoefficient/MachRegion2/Ccdaib/Ccdaib_ ==
  angleOfAttack_deg : Inport
  dAI : Inport  Port=2
  angleOfSideslip_deg : Inport  Port=3
  tflow : Inport  Port=4
  eieff : Inport  Port=5
  Abs : Abs
  Abs1 : Abs
  Abs2 : Abs
  CCDABAL_ALFA : Lookup_n-D  NumberOfTableDimensions=1  BreakpointsForDimension1=admireDB.aerodata_asym_ext.CCDABAL.breakpoints.ALFA  BreakpointsForDimension3=[5, 7]  Table=admireDB.aerodata_asym_ext.CCDABAL.newTable  ExtrapMethod=Clip  InternalRulePriority=Speed  RndMeth=Simplest  InputSameDT=on
  Constant : Constant  Value=1/30
  Constant1 : Constant  Value=1/20
  Product : Product
  Product1 : Product
  Product2 : Product  Inputs=5
  Ccdaib : Outport
  wires:
  Product2/1 -> Ccdaib/1
  angleOfSideslip_deg/1 -> Abs2/1
  angleOfAttack_deg/1 -> Abs/1
  Abs/1 -> CCDABAL_ALFA/1
  dAI/1 -> Abs1/1
  Abs1/1 -> Product/1
  Constant/1 -> Product/2
  Constant1/1 -> Product1/2
  Abs2/1 -> Product1/1
  tflow/1 -> Product2/2
  eieff/1 -> Product2/4
  CCDABAL_ALFA/1 -> Product2/1
  Product/1 -> Product2/3
  Product1/1 -> Product2/5

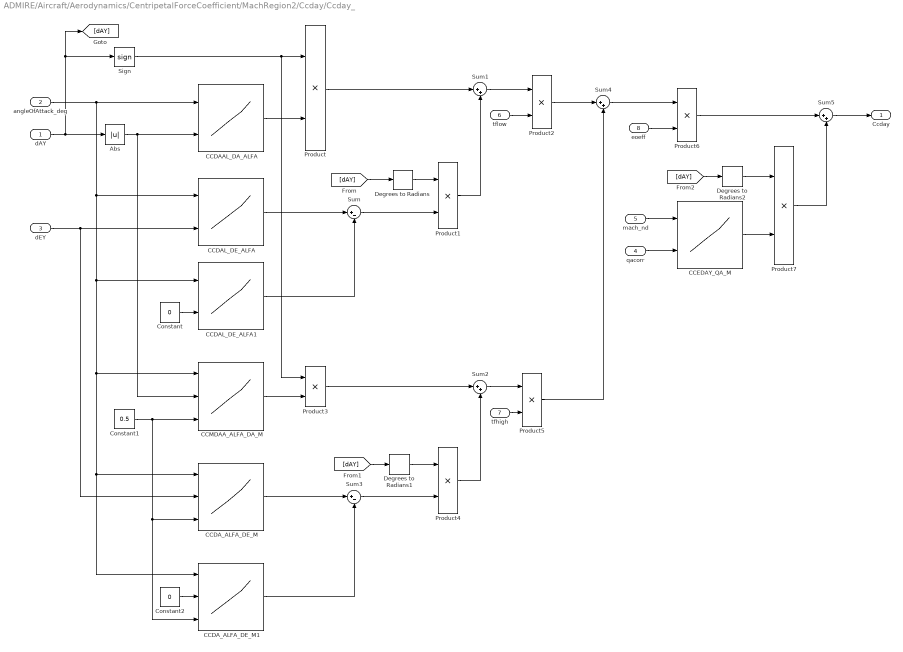
== system ADMIRE/Aircraft/Aerodynamics/CentripetalForceCoefficient/MachRegion2/Ccday/Ccday_ ==
  dAY : Inport
  angleOfAttack_deg : Inport  Port=2
  dEY : Inport  Port=3
  qacorr : Inport  Port=4
  mach_nd : Inport  Port=5
  tflow : Inport  Port=6
  tfhigh : Inport  Port=7
  eoeff : Inport  Port=8
  Abs : Abs
  CCDAAL_DA_ALFA : Lookup_n-D  BreakpointsForDimension1=admireDB.aerodata_asym_ext.CCDAAL.breakpoints.ALFA  BreakpointsForDimension2=admireDB.aerodata_asym_ext.CCDAAL.breakpoints.DA  BreakpointsForDimension3=[5, 7]  Table=admireDB.aerodata_asym_ext.CCDAAL.newTable  ExtrapMethod=Clip  InternalRulePriority=Speed  RndMeth=Simplest  InputSameDT=on
      settings: InputPortMap=u0,u1
  CCDAL_DE_ALFA : Lookup_n-D  BreakpointsForDimension1=admireDB.aerodata_asym_ext.CCDAL.breakpoints.ALFA  BreakpointsForDimension2=admireDB.aerodata_asym_ext.CCDAL.breakpoints.DE  BreakpointsForDimension3=[5, 7]  Table=admireDB.aerodata_asym_ext.CCDAL.newTable  ExtrapMethod=Clip  InternalRulePriority=Speed  RndMeth=Simplest  InputSameDT=on
      settings: InputPortMap=u0,u1
  CCDAL_DE_ALFA1 : Lookup_n-D  BreakpointsForDimension1=admireDB.aerodata_asym_ext.CCDAL.breakpoints.ALFA  BreakpointsForDimension2=admireDB.aerodata_asym_ext.CCDAL.breakpoints.DE  BreakpointsForDimension3=[5, 7]  Table=admireDB.aerodata_asym_ext.CCDAL.newTable  ExtrapMethod=Clip  InternalRulePriority=Speed  RndMeth=Simplest  InputSameDT=on
      settings: InputPortMap=u0,u1
  CCDA_ALFA_DE_M : Lookup_n-D  NumberOfTableDimensions=3  BreakpointsForDimension1=admireDB.aerodata_asym_ext.CCDA.breakpoints.ALFA  BreakpointsForDimension2=admireDB.aerodata_asym_ext.CCDA.breakpoints.DE  BreakpointsForDimension3=admireDB.aerodata_asym_ext.CCDA.breakpoints.M  Table=admireDB.aerodata_asym_ext.CCDA.newTable  ExtrapMethod=Clip  InternalRulePriority=Speed  RndMeth=Simplest  InputSameDT=on
      settings: InputPortMap=u0,u1,u2
  CCDA_ALFA_DE_M1 : Lookup_n-D  NumberOfTableDimensions=3  BreakpointsForDimension1=admireDB.aerodata_asym_ext.CCDA.breakpoints.ALFA  BreakpointsForDimension2=admireDB.aerodata_asym_ext.CCDA.breakpoints.DE  BreakpointsForDimension3=admireDB.aerodata_asym_ext.CCDA.breakpoints.M  Table=admireDB.aerodata_asym_ext.CCDA.newTable  ExtrapMethod=Clip  InternalRulePriority=Speed  RndMeth=Simplest  InputSameDT=on
      settings: InputPortMap=u0,u1,u2
  CCEDAY_QA_M : Lookup_n-D  BreakpointsForDimension1=admireDB.aerodata_asym_ext.CCEDAY.breakpoints.M  BreakpointsForDimension2=admireDB.aerodata_asym_ext.CCEDAY.breakpoints.QA  BreakpointsForDimension3=[5, 7]  Table=admireDB.aerodata_asym_ext.CCEDAY.newTable  ExtrapMethod=Clip  InternalRulePriority=Speed  RndMeth=Simplest  InputSameDT=on
      settings: InputPortMap=u0,u1
  CCMDAA_ALFA_DA_M : Lookup_n-D  NumberOfTableDimensions=3  BreakpointsForDimension1=admireDB.aerodata_asym_ext.CCMDAA.breakpoints.ALFA  BreakpointsForDimension2=admireDB.aerodata_asym_ext.CCMDAA.breakpoints.DA  BreakpointsForDimension3=admireDB.aerodata_asym_ext.CCMDAA.breakpoints.M  Table=admireDB.aerodata_asym_ext.CCMDAA.newTable  ExtrapMethod=Clip  InternalRulePriority=Speed  RndMeth=Simplest  InputSameDT=on
      settings: InputPortMap=u0,u1,u2
  Constant : Constant  Value=0
  Constant1 : Constant  Value=0.5
  Constant2 : Constant  Value=0
  Degrees to Radians : simulink_extras/Transformations/Degrees to Radians
  Degrees to Radians1 : simulink_extras/Transformations/Degrees to Radians
  Degrees to Radians2 : simulink_extras/Transformations/Degrees to Radians
  Product{,1..7} (8 alike) : Product
  Sign : Signum
  Sum : Sum  Inputs=|+-
  Sum{1..2,4..5} (4 alike) : Sum  Inputs=|++
  Sum3 : Sum  Inputs=|+-
  Ccday : Outport
  wires:
  Sum5/1 -> Ccday/1
  Degrees to Radians2/1 -> Product7/1
  [dAY] -> Degrees to Radians2/1
  CCDA_ALFA_DE_M1/1 -> Sum3/2
  Constant2/1 -> CCDA_ALFA_DE_M1/2
  CCDAL_DE_ALFA1/1 -> Sum/2
  Constant/1 -> CCDAL_DE_ALFA1/2
  dEY/1 -> CCDA_ALFA_DE_M/2, CCDAL_DE_ALFA/2
  angleOfAttack_deg/1 -> CCDAL_DE_ALFA/1, CCDAL_DE_ALFA1/1, CCDA_ALFA_DE_M1/1, CCDA_ALFA_DE_M/1, CCMDAA_ALFA_DA_M/1, CCDAAL_DA_ALFA/1
  dAY/1 -> Abs/1, [dAY], Sign/1
  CCDAAL_DA_ALFA/1 -> Product/2
  Sign/1 -> Product/1, Product3/1
  CCDAL_DE_ALFA/1 -> Sum/1
  [dAY] -> Degrees to Radians/1
  Degrees to Radians/1 -> Product1/1
  Sum/1 -> Product1/2
  Product/1 -> Sum1/1
  Product1/1 -> Sum1/2
  Sum1/1 -> Product2/1
  tflow/1 -> Product2/2
  Abs/1 -> CCDAAL_DA_ALFA/2, CCMDAA_ALFA_DA_M/2
  Constant1/1 -> CCDA_ALFA_DE_M1/3, CCDA_ALFA_DE_M/3, CCMDAA_ALFA_DA_M/3
  CCMDAA_ALFA_DA_M/1 -> Product3/2
  Product3/1 -> Sum2/1
  Sum3/1 -> Product4/2
  CCDA_ALFA_DE_M/1 -> Sum3/1
  [dAY] -> Degrees to Radians1/1
  Degrees to Radians1/1 -> Product4/1
  Product4/1 -> Sum2/2
  Sum2/1 -> Product5/1
  tfhigh/1 -> Product5/2
  Product2/1 -> Sum4/1
  Product5/1 -> Sum4/2
  eoeff/1 -> Product6/2
  Sum4/1 -> Product6/1
  Product6/1 -> Sum5/1
  mach_nd/1 -> CCEDAY_QA_M/1
  qacorr/1 -> CCEDAY_QA_M/2
  CCEDAY_QA_M/1 -> Product7/2
  Product7/1 -> Sum5/2

== system ADMIRE/Aircraft/Aerodynamics/CentripetalForceCoefficient/MachRegion2/Ccdayb/Ccdayb_ ==
  angleOfAttack_deg : Inport
  dAY : Inport  Port=2
  angleOfSideslip_deg : Inport  Port=3
  tflow : Inport  Port=4
  eoeff : Inport  Port=5
  Abs : Abs
  Abs1 : Abs
  Abs2 : Abs
  CCDABAL_ALFA : Lookup_n-D  NumberOfTableDimensions=1  BreakpointsForDimension1=admireDB.aerodata_asym_ext.CCDABAL.breakpoints.ALFA  BreakpointsForDimension3=[5, 7]  Table=admireDB.aerodata_asym_ext.CCDABAL.newTable  ExtrapMethod=Clip  InternalRulePriority=Speed  RndMeth=Simplest  InputSameDT=on
  Constant : Constant  Value=1/30
  Constant1 : Constant  Value=1/20
  Product : Product
  Product1 : Product
  Product2 : Product  Inputs=5
  Ccdaib : Outport
  wires:
  Product2/1 -> Ccdaib/1
  Product1/1 -> Product2/5
  Product/1 -> Product2/3
  CCDABAL_ALFA/1 -> Product2/1
  eoeff/1 -> Product2/4
  tflow/1 -> Product2/2
  Abs2/1 -> Product1/1
  Constant1/1 -> Product1/2
  Constant/1 -> Product/2
  Abs1/1 -> Product/1
  dAY/1 -> Abs1/1
  Abs/1 -> CCDABAL_ALFA/1
  angleOfAttack_deg/1 -> Abs/1
  angleOfSideslip_deg/1 -> Abs2/1

== system ADMIRE/Aircraft/Aerodynamics/CentripetalForceCoefficient/MachRegion2/Ccdna/Ccdna_ ==
  dNE : Inport
  angleOfAttack_deg : Inport  Port=2
  tflow : Inport  Port=3
  tfhigh : Inport  Port=4
  dNA : Inport  Port=5
  CCDNAAL_DNE_ALFA : Lookup_n-D  BreakpointsForDimension1=admireDB.aerodata_asym_ext.CCDNAAL.breakpoints.ALFA  BreakpointsForDimension2=admireDB.aerodata_asym_ext.CCDNAAL.breakpoints.DNE  BreakpointsForDimension3=[5, 7]  Table=admireDB.aerodata_asym_ext.CCDNAAL.newTable  ExtrapMethod=Clip  InternalRulePriority=Speed  RndMeth=Simplest  InputSameDT=on
      settings: InputPortMap=u0,u1
  CCDNAAM_ALFA_M : Lookup_n-D  BreakpointsForDimension1=admireDB.aerodata_asym_ext.CCDNAAM.breakpoints.M  BreakpointsForDimension2=admireDB.aerodata_asym_ext.CCDNAAM.breakpoints.ALFA  BreakpointsForDimension3=[5, 7]  Table=admireDB.aerodata_asym_ext.CCDNAAM.newTable  ExtrapMethod=Clip  InternalRulePriority=Speed  RndMeth=Simplest  InputSameDT=on
      settings: InputPortMap=u0,u1
  Constant : Constant  Value=0.5
  Degrees to Radians : simulink_extras/Transformations/Degrees to Radians
  Product : Product
  Product1 : Product
  Product2 : Product
  Sum : Sum  Inputs=|++
  Ccdna : Outport
  wires:
  dNE/1 -> CCDNAAL_DNE_ALFA/2
  angleOfAttack_deg/1 -> CCDNAAM_ALFA_M/2, CCDNAAL_DNE_ALFA/1
  tflow/1 -> Product/2
  CCDNAAL_DNE_ALFA/1 -> Product/1
  Constant/1 -> CCDNAAM_ALFA_M/1
  CCDNAAM_ALFA_M/1 -> Product1/2
  tfhigh/1 -> Product1/1
  Product/1 -> Sum/1
  Product1/1 -> Sum/2
  dNA/1 -> Degrees to Radians/1
  Degrees to Radians/1 -> Product2/2
  Sum/1 -> Product2/1
  Product2/1 -> Ccdna/1

== system ADMIRE/Aircraft/Aerodynamics/CentripetalForceCoefficient/MachRegion2/Ccdr/Ccdr_ ==
  angleOfAttack_deg : Inport
  dR : Inport  Port=2
  angleOfSideslip_deg : Inport  Port=3
  tflow : Inport  Port=4
  tfhigh : Inport  Port=5
  qacorr : Inport  Port=6
  mach_nd : Inport  Port=7
  Abs : Abs
  CCBDRAL_ALFA_DR_BETA : Lookup_n-D  NumberOfTableDimensions=3  BreakpointsForDimension1=admireDB.aerodata_asym_ext.CCBDRAL.breakpoints.ALFA  BreakpointsForDimension2=admireDB.aerodata_asym_ext.CCBDRAL.breakpoints.DR  BreakpointsForDimension3=admireDB.aerodata_asym_ext.CCBDRAL.breakpoints.BETA  Table=admireDB.aerodata_asym_ext.CCBDRAL.newTable  ExtrapMethod=Clip  InternalRulePriority=Speed  RndMeth=Simplest  InputSameDT=on
      settings: InputPortMap=u0,u1,u2
  CCDRAM_ALFA_M : Lookup_n-D  BreakpointsForDimension1=admireDB.aerodata_asym_ext.CCDRAM.breakpoints.M  BreakpointsForDimension2=admireDB.aerodata_asym_ext.CCDRAM.breakpoints.ALFA  BreakpointsForDimension3=[5, 7]  Table=admireDB.aerodata_asym_ext.CCDRAM.newTable  ExtrapMethod=Clip  InternalRulePriority=Speed  RndMeth=Simplest  InputSameDT=on
      settings: InputPortMap=u0,u1
  CCEDR_QA_M : Lookup_n-D  BreakpointsForDimension1=admireDB.aerodata_asym_ext.CCEDR.breakpoints.M  BreakpointsForDimension2=admireDB.aerodata_asym_ext.CCEDR.breakpoints.QA  BreakpointsForDimension3=[5, 7]  Table=admireDB.aerodata_asym_ext.CCEDR.newTable  ExtrapMethod=Clip  InternalRulePriority=Speed  RndMeth=Simplest  InputSameDT=on
      settings: InputPortMap=u0,u1
  Constant : Constant  Value=0.5
  Degrees to Radians : simulink_extras/Transformations/Degrees to Radians
  Product : Product
  Product1 : Product  Inputs=3
  Product2 : Product
  Sum : Sum  Inputs=|++
  Ccdr : Outport
  wires:
  Product2/1 -> Ccdr/1
  angleOfAttack_deg/1 -> CCBDRAL_ALFA_DR_BETA/1, CCDRAM_ALFA_M/2
  dR/1 -> Degrees to Radians/1, CCBDRAL_ALFA_DR_BETA/2
  angleOfSideslip_deg/1 -> Abs/1
  CCBDRAL_ALFA_DR_BETA/1 -> Product/1
  tflow/1 -> Product/2
  Product/1 -> Sum/1
  Constant/1 -> CCDRAM_ALFA_M/1
  tfhigh/1 -> Product1/3
  CCDRAM_ALFA_M/1 -> Product1/2
  Degrees to Radians/1 -> Product1/1
  qacorr/1 -> CCEDR_QA_M/2
  mach_nd/1 -> CCEDR_QA_M/1
  CCEDR_QA_M/1 -> Product2/2
  Product1/1 -> Sum/2
  Sum/1 -> Product2/1
  Abs/1 -> CCBDRAL_ALFA_DR_BETA/3

== system ADMIRE/Aircraft/Aerodynamics/CentripetalForceCoefficient/MachRegion2/Ccp/Ccp_ ==
  angleOfAttack_deg : Inport
  tflow : Inport  Port=2
  pc : Inport  Port=3
  tfhigh : Inport  Port=4
  CCPAL_ALFA : Lookup_n-D  NumberOfTableDimensions=1  BreakpointsForDimension1=admireDB.aerodata_asym_ext.CCPAL.breakpoints.ALFA  BreakpointsForDimension3=[5, 7]  Table=admireDB.aerodata_asym_ext.CCPAL.newTable  ExtrapMethod=Clip  InternalRulePriority=Speed  RndMeth=Simplest  InputSameDT=on
  CCPAM_ALFA_M : Lookup_n-D  BreakpointsForDimension1=admireDB.aerodata_asym_ext.CCPAM.breakpoints.M  BreakpointsForDimension2=admireDB.aerodata_asym_ext.CCPAM.breakpoints.ALFA  BreakpointsForDimension3=[5, 7]  Table=admireDB.aerodata_asym_ext.CCPAM.newTable  ExtrapMethod=Clip  InternalRulePriority=Speed  RndMeth=Simplest  InputSameDT=on
      settings: InputPortMap=u0,u1
  Constant : Constant  Value=0.5
  Product : Product
  Product1 : Product
  Product2 : Product
  Sum : Sum  Inputs=|++
  Ccp : Outport
  wires:
  angleOfAttack_deg/1 -> CCPAL_ALFA/1, CCPAM_ALFA_M/2
  tflow/1 -> Product/2
  CCPAL_ALFA/1 -> Product/1
  Product/1 -> Sum/1
  Constant/1 -> CCPAM_ALFA_M/1
  CCPAM_ALFA_M/1 -> Product1/2
  tfhigh/1 -> Product1/1
  Product1/1 -> Sum/2
  Sum/1 -> Product2/1
  pc/1 -> Product2/2
  Product2/1 -> Ccp/1

== system ADMIRE/Aircraft/Aerodynamics/CentripetalForceCoefficient/MachRegion2/Ccpbeta/Ccpbeta_ ==
  angleOfSideslip_deg : Inport
  angleOfAttack_deg : Inport  Port=2
  tflow : Inport  Port=3
  pc : Inport  Port=4
  Abs : Abs
  CCPBA_BETA_ALFA : Lookup_n-D  BreakpointsForDimension1=admireDB.aerodata_asym_ext.CCPBA.breakpoints.ALFA  BreakpointsForDimension2=admireDB.aerodata_asym_ext.CCPBA.breakpoints.BETA  BreakpointsForDimension3=[5, 7]  Table=admireDB.aerodata_asym_ext.CCPBA.newTable  ExtrapMethod=Clip  InternalRulePriority=Speed  RndMeth=Simplest  InputSameDT=on
      settings: InputPortMap=u0,u1
  Product : Product  Inputs=3
  Ccpbeta : Outport
  wires:
  CCPBA_BETA_ALFA/1 -> Product/1
  tflow/1 -> Product/2
  angleOfAttack_deg/1 -> CCPBA_BETA_ALFA/1
  angleOfSideslip_deg/1 -> Abs/1
  Abs/1 -> CCPBA_BETA_ALFA/2
  pc/1 -> Product/3
  Product/1 -> Ccpbeta/1

== system ADMIRE/Aircraft/Aerodynamics/CentripetalForceCoefficient/MachRegion2/Ccr/Ccr_ ==
  dN : Inport
  angleOfAttack_deg : Inport  Port=2
  tflow : Inport  Port=3
  tfhigh : Inport  Port=4
  rc : Inport  Port=5
  mach_nd : Inport  Port=6
  qacorr : Inport  Port=7
  CCER_M_QA : Lookup_n-D  BreakpointsForDimension1=admireDB.aerodata_asym_ext.CCER.breakpoints.QA  BreakpointsForDimension2=admireDB.aerodata_asym_ext.CCER.breakpoints.M  BreakpointsForDimension3=[5, 7]  Table=admireDB.aerodata_asym_ext.CCER.newTable  ExtrapMethod=Clip  InternalRulePriority=Speed  RndMeth=Simplest  InputSameDT=on
      settings: InputPortMap=u0,u1
  CCRAL_DNV_ALFA : Lookup_n-D  BreakpointsForDimension1=admireDB.aerodata_asym_ext.CCRAL.breakpoints.ALFA  BreakpointsForDimension2=admireDB.aerodata_asym_ext.CCRAL.breakpoints.DNV  BreakpointsForDimension3=[5, 7]  Table=admireDB.aerodata_asym_ext.CCRAL.newTable  ExtrapMethod=Clip  InternalRulePriority=Speed  RndMeth=Simplest  InputSameDT=on
      settings: InputPortMap=u0,u1
  CCRM_M : Lookup_n-D  NumberOfTableDimensions=1  BreakpointsForDimension1=admireDB.aerodata_asym_ext.CCRM.breakpoints.M  BreakpointsForDimension3=[5, 7]  Table=admireDB.aerodata_asym_ext.CCRM.newTable  ExtrapMethod=Clip  InternalRulePriority=Speed  RndMeth=Simplest  InputSameDT=on
  Constant : Constant  Value=0.5
  Product{,1..3} (4 alike) : Product
  Sum : Sum  Inputs=|++
  Ccr : Outport
  wires:
  Product2/1 -> Product3/1
  rc/1 -> Product2/2
  Sum/1 -> Product2/1
  Product1/1 -> Sum/2
  tfhigh/1 -> Product1/1
  CCRM_M/1 -> Product1/2
  Constant/1 -> CCRM_M/1
  Product/1 -> Sum/1
  CCRAL_DNV_ALFA/1 -> Product/1
  tflow/1 -> Product/2
  angleOfAttack_deg/1 -> CCRAL_DNV_ALFA/1
  dN/1 -> CCRAL_DNV_ALFA/2
  Product3/1 -> Ccr/1
  CCER_M_QA/1 -> Product3/2
  mach_nd/1 -> CCER_M_QA/2
  qacorr/1 -> CCER_M_QA/1
